simulink model "MultiBody2024bfinal"  (R2024b)
settings: Solver=ode45  StartTime=0.0  StopTime=5  FixedStep=0.001  RelTol=1e-3  AbsTol=1e-3  EnableMultiTasking=on
InitFcn:
  | contact_damping = 1e4;
  | contact_stiffness = 1e6;
values from neighbouring files (symbols this model uses):
  Angle = [30 30 0]    [main_SuperTwistingSMC2.m]
  Height = -(1.9 + i)    (= -5.9)    [main_SuperTwistingSMC2.m]
  i = 4    [main_SuperTwistingSMC2.m]
  nt = n_t(i)    [main_SuperTwistingSMC2.m]
  TM = TMM(i)    [main_SuperTwistingSMC2.m]
  TotalWeight = TotalWeightmb(i)    [main_SuperTwistingSMC2.m]
undefined symbols (not defined in the file or in its folder): X, Y, Z
libraries: sm_lib x207, nesl_utility x73, sharedtransform x6, simulink_extras x4
(part 7 of 7)

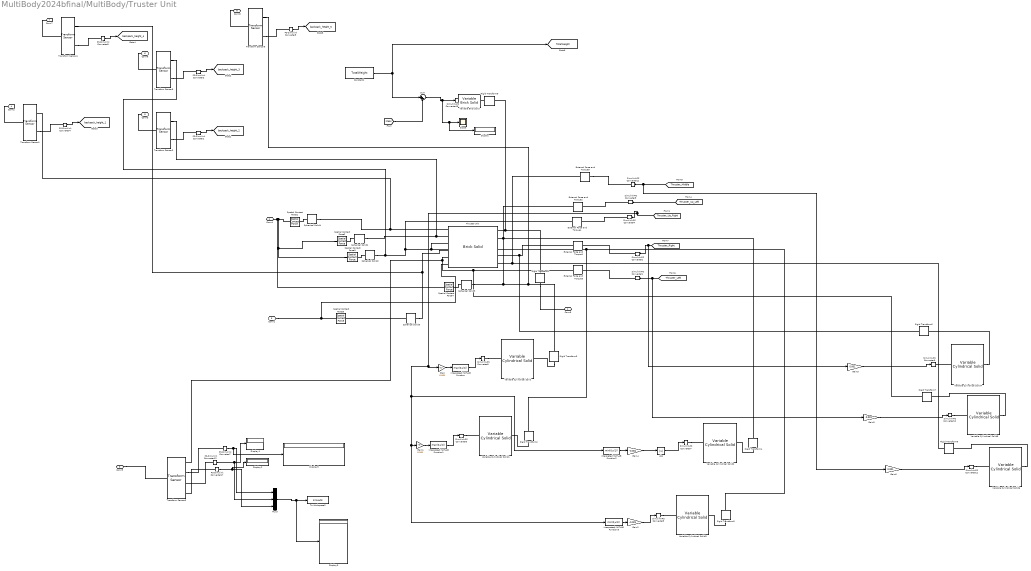
== system MultiBody2024bfinal/MultiBody/Truster Unit ==
  Abs : Abs  SaturateOnIntegerOverflow=off
  Constant1 : Constant  Value=TotalWeight
  Display{,1..3,5} (5 alike) : Display
  External Force and Torque1 : sm_lib/Forces and Torques/External Force and Torque  EnableForceX=off  EnableForceY=on  EnableForceZ=off  EnableForce=off  ForceResolutionFrame=AttachedFrame  EnableTorqueX=off  EnableTorqueY=off  EnableTorqueZ=off  EnableTorque=off  TorqueResolutionFrame=AttachedFrame
  External Force and Torque2 : sm_lib/Forces and Torques/External Force and Torque  EnableForceX=on  EnableForceY=off  EnableForceZ=off  EnableForce=off  ForceResolutionFrame=AttachedFrame  EnableTorqueX=off  EnableTorqueY=off  EnableTorqueZ=off  EnableTorque=off  TorqueResolutionFrame=AttachedFrame
  External Force and Torque3 : sm_lib/Forces and Torques/External Force and Torque  EnableForceX=off  EnableForceY=on  EnableForceZ=off  EnableForce=off  ForceResolutionFrame=AttachedFrame  EnableTorqueX=off  EnableTorqueY=off  EnableTorqueZ=off  EnableTorque=off  TorqueResolutionFrame=AttachedFrame
  External Force and Torque4 : sm_lib/Forces and Torques/External Force and Torque  EnableForceX=on  EnableForceY=off  EnableForceZ=off  EnableForce=off  ForceResolutionFrame=AttachedFrame  EnableTorqueX=off  EnableTorqueY=off  EnableTorqueZ=off  EnableTorque=off  TorqueResolutionFrame=AttachedFrame
  External Force and Torque5 : sm_lib/Forces and Torques/External Force and Torque  EnableForceX=off  EnableForceY=on  EnableForceZ=off  EnableForce=off  ForceResolutionFrame=AttachedFrame  EnableTorqueX=off  EnableTorqueY=off  EnableTorqueZ=off  EnableTorque=off  TorqueResolutionFrame=AttachedFrame
  Gain{,1,3,5..6} (5 alike) : Gain  Gain=0.001
  Gain2 : Gain  Gain=-0.001
  Gain4 : Gain  Gain=-0.001
  Interpreted MATLAB Function : MATLABFcn  MATLABFcn=max(0,u(1))
  Interpreted MATLAB Function1 : MATLABFcn  MATLABFcn=max(0,u(1))
  Interpreted MATLAB Function2 : MATLABFcn  MATLABFcn=min(0,u(1))
  Interpreted MATLAB Function3 : MATLABFcn  MATLABFcn=min(0,u(1))
  Mux3 : Mux  Inputs=3
  PS-Simulink Converter{1..5,7,12,17} (8 alike) : nesl_utility/PS-Simulink Converter  PhysicalDomain=network_engine_domain  SubClassName=ps_output  LeftPortType=input  RightPortType=output  PseudoPeriodic=off  Frequencies=[]  VectorFormat=inherit  Unit=inherit  AffineConversion=off
  Rigid Transform1 : sm_lib/Frames and Transforms/Rigid Transform  RotationMethod=None  FollAlignAxisA=+X  BaseAlignAxisA=+Y  FollAlignAxisB=+Y  BaseAlignAxisB=+Z  RotationStandardAxis=+Z  RotationAngle=0.0  RotationAngleUnits=deg  RotationArbitraryAxis=[0 0 1]  RotationSequenceAxes=FollowerAxes  RotationSequence=XYX  RotationSequenceAngles=[0 0 0]  RotationSequenceAnglesUnits=deg  RotationMatrix=[1 0 0; 0 1 0; 0 0 1]  Quaternion=[1 0 0 0]  TranslationMethod=Cartesian  TranslationCartesianOffset=[-0.17 0.17 1.903701373840161e-04]  TranslationCartesianOffsetUnits=m  TranslationStandardAxis=-X  TranslationStandardOffset=0.16  TranslationStandardOffsetUnits=m  TranslationROffset=0  TranslationROffsetUnits=m  TranslationThetaOffset=0  TranslationThetaOffsetUnits=deg  TranslationZOffset=0  TranslationZOffsetUnits=m
  Rigid Transform2 : sm_lib/Frames and Transforms/Rigid Transform  RotationMethod=StandardAxis  FollAlignAxisA=+X  BaseAlignAxisA=+Y  FollAlignAxisB=+Y  BaseAlignAxisB=+Z  RotationStandardAxis=+Y  RotationAngle=90  RotationAngleUnits=deg  RotationArbitraryAxis=[0 0 1]  RotationSequenceAxes=FollowerAxes  RotationSequence=XYX  RotationSequenceAngles=[0 0 0]  RotationSequenceAnglesUnits=deg  RotationMatrix=[1 0 0; 0 1 0; 0 0 1]  Quaternion=[1 0 0 0]  TranslationMethod=None  TranslationCartesianOffset=[-0.17 0.17 0]  TranslationCartesianOffsetUnits=m  TranslationStandardAxis=-X  TranslationStandardOffset=0.16  TranslationStandardOffsetUnits=m  TranslationROffset=0  TranslationROffsetUnits=m  TranslationThetaOffset=0  TranslationThetaOffsetUnits=deg  TranslationZOffset=0  TranslationZOffsetUnits=m
  Rigid Transform3 : sm_lib/Frames and Transforms/Rigid Transform  RotationMethod=StandardAxis  FollAlignAxisA=+X  BaseAlignAxisA=+Y  FollAlignAxisB=+Y  BaseAlignAxisB=+Z  RotationStandardAxis=+Y  RotationAngle=90  RotationAngleUnits=deg  RotationArbitraryAxis=[0 0 1]  RotationSequenceAxes=FollowerAxes  RotationSequence=XYX  RotationSequenceAngles=[0 0 0]  RotationSequenceAnglesUnits=deg  RotationMatrix=[1 0 0; 0 1 0; 0 0 1]  Quaternion=[1 0 0 0]  TranslationMethod=None  TranslationCartesianOffset=[-0.17 0.17 0]  TranslationCartesianOffsetUnits=m  TranslationStandardAxis=-X  TranslationStandardOffset=0.16  TranslationStandardOffsetUnits=m  TranslationROffset=0  TranslationROffsetUnits=m  TranslationThetaOffset=0  TranslationThetaOffsetUnits=deg  TranslationZOffset=0  TranslationZOffsetUnits=m
  Rigid Transform4 : sm_lib/Frames and Transforms/Rigid Transform  RotationMethod=StandardAxis  FollAlignAxisA=+X  BaseAlignAxisA=+Y  FollAlignAxisB=+Y  BaseAlignAxisB=+Z  RotationStandardAxis=+Y  RotationAngle=-90  RotationAngleUnits=deg  RotationArbitraryAxis=[0 0 1]  RotationSequenceAxes=FollowerAxes  RotationSequence=XYX  RotationSequenceAngles=[0 0 0]  RotationSequenceAnglesUnits=deg  RotationMatrix=[1 0 0; 0 1 0; 0 0 1]  Quaternion=[1 0 0 0]  TranslationMethod=None  TranslationCartesianOffset=[-0.17 0.17 0]  TranslationCartesianOffsetUnits=m  TranslationStandardAxis=-X  TranslationStandardOffset=0.16  TranslationStandardOffsetUnits=m  TranslationROffset=0  TranslationROffsetUnits=m  TranslationThetaOffset=0  TranslationThetaOffsetUnits=deg  TranslationZOffset=0  TranslationZOffsetUnits=m
  Rigid Transform5 : sm_lib/Frames and Transforms/Rigid Transform  RotationMethod=StandardAxis  FollAlignAxisA=+X  BaseAlignAxisA=+Y  FollAlignAxisB=+Y  BaseAlignAxisB=+Z  RotationStandardAxis=+Y  RotationAngle=-90  RotationAngleUnits=deg  RotationArbitraryAxis=[0 0 1]  RotationSequenceAxes=FollowerAxes  RotationSequence=XYX  RotationSequenceAngles=[0 0 0]  RotationSequenceAnglesUnits=deg  RotationMatrix=[1 0 0; 0 1 0; 0 0 1]  Quaternion=[1 0 0 0]  TranslationMethod=None  TranslationCartesianOffset=[-0.17 0.17 0]  TranslationCartesianOffsetUnits=m  TranslationStandardAxis=-X  TranslationStandardOffset=0.16  TranslationStandardOffsetUnits=m  TranslationROffset=0  TranslationROffsetUnits=m  TranslationThetaOffset=0  TranslationThetaOffsetUnits=deg  TranslationZOffset=0  TranslationZOffsetUnits=m
  Rigid Transform6 : sm_lib/Frames and Transforms/Rigid Transform  RotationMethod=StandardAxis  FollAlignAxisA=+X  BaseAlignAxisA=+Y  FollAlignAxisB=+Y  BaseAlignAxisB=+Z  RotationStandardAxis=+X  RotationAngle=-90  RotationAngleUnits=deg  RotationArbitraryAxis=[0 0 1]  RotationSequenceAxes=FollowerAxes  RotationSequence=XYX  RotationSequenceAngles=[0 0 0]  RotationSequenceAnglesUnits=deg  RotationMatrix=[1 0 0; 0 1 0; 0 0 1]  Quaternion=[1 0 0 0]  TranslationMethod=None  TranslationCartesianOffset=[-0.17 0.17 0]  TranslationCartesianOffsetUnits=m  TranslationStandardAxis=-X  TranslationStandardOffset=0.16  TranslationStandardOffsetUnits=m  TranslationROffset=0  TranslationROffsetUnits=m  TranslationThetaOffset=0  TranslationThetaOffsetUnits=deg  TranslationZOffset=0  TranslationZOffsetUnits=m
  Rigid Transform7 : sm_lib/Frames and Transforms/Rigid Transform  RotationMethod=StandardAxis  FollAlignAxisA=+X  BaseAlignAxisA=+Y  FollAlignAxisB=+Y  BaseAlignAxisB=+Z  RotationStandardAxis=+X  RotationAngle=-90  RotationAngleUnits=deg  RotationArbitraryAxis=[0 0 1]  RotationSequenceAxes=FollowerAxes  RotationSequence=XYX  RotationSequenceAngles=[0 0 0]  RotationSequenceAnglesUnits=deg  RotationMatrix=[1 0 0; 0 1 0; 0 0 1]  Quaternion=[1 0 0 0]  TranslationMethod=None  TranslationCartesianOffset=[-0.17 0.17 0]  TranslationCartesianOffsetUnits=m  TranslationStandardAxis=-X  TranslationStandardOffset=0.16  TranslationStandardOffsetUnits=m  TranslationROffset=0  TranslationROffsetUnits=m  TranslationThetaOffset=0  TranslationThetaOffsetUnits=deg  TranslationZOffset=0  TranslationZOffsetUnits=m
  Rigid Transform8 : sm_lib/Frames and Transforms/Rigid Transform  RotationMethod=StandardAxis  FollAlignAxisA=+X  BaseAlignAxisA=+Y  FollAlignAxisB=+Y  BaseAlignAxisB=+Z  RotationStandardAxis=+X  RotationAngle=-90  RotationAngleUnits=deg  RotationArbitraryAxis=[0 0 1]  RotationSequenceAxes=FollowerAxes  RotationSequence=XYX  RotationSequenceAngles=[0 0 0]  RotationSequenceAnglesUnits=deg  RotationMatrix=[1 0 0; 0 1 0; 0 0 1]  Quaternion=[1 0 0 0]  TranslationMethod=None  TranslationCartesianOffset=[-0.17 0.17 0]  TranslationCartesianOffsetUnits=m  TranslationStandardAxis=-X  TranslationStandardOffset=0.16  TranslationStandardOffsetUnits=m  TranslationROffset=0  TranslationROffsetUnits=m  TranslationThetaOffset=0  TranslationThetaOffsetUnits=deg  TranslationZOffset=0  TranslationZOffsetUnits=m
  Rigid Transform9 : sm_lib/Frames and Transforms/Rigid Transform  RotationMethod=None  FollAlignAxisA=+X  BaseAlignAxisA=+Y  FollAlignAxisB=+Y  BaseAlignAxisB=+Z  RotationStandardAxis=+Z  RotationAngle=0.0  RotationAngleUnits=deg  RotationArbitraryAxis=[0 0 1]  RotationSequenceAxes=FollowerAxes  RotationSequence=XYX  RotationSequenceAngles=[0 0 0]  RotationSequenceAnglesUnits=deg  RotationMatrix=[1 0 0; 0 1 0; 0 0 1]  Quaternion=[1 0 0 0]  TranslationMethod=Cartesian  TranslationCartesianOffset=[0 0 -0.33/2]  TranslationCartesianOffsetUnits=m  TranslationStandardAxis=-X  TranslationStandardOffset=0.16  TranslationStandardOffsetUnits=m  TranslationROffset=0  TranslationROffsetUnits=m  TranslationThetaOffset=0  TranslationThetaOffsetUnits=deg  TranslationZOffset=0  TranslationZOffsetUnits=m
  Scope : Scope
  Simulink-PS Converter{1..13} (13 alike) : nesl_utility/Simulink-PS Converter  PhysicalDomain=network_engine_domain  SubClassName=ps_input  LeftPortType=input  RightPortType=output  PseudoPeriodic=off  Frequencies=[]  NoiseDistribution=none  NoiseParameters=[]  Unit=1  AffineConversion=off  FilteringAndDerivatives=provide  SimscapeFilterOrder=1  InputFilterTimeConstant=0.001  UdotUserProvided=0
  Spatial Contact Force{1..5} (5 alike) : sm_lib/Forces and Torques/Spatial Contact Force  NormalForceType=SmoothSpringDamper  NormalStiffness=contact_stiffness  NormalStiffnessUnits=N/m  NormalDamping=contact_damping  NormalDampingUnits=N/(m/s)  NormalTransitionRegionWidth=1e-4  NormalTransitionRegionWidthUnits=m  FrictionType=SmoothStickSlip  CoefficientOfStaticFriction=0.5  CoefficientOfDynamicFriction=0.3  FrictionalCriticalVelocity=1e-3  FrictionalCriticalVelocityUnits=m/s  SenseContactSignal=off  SensePenetrationDepth=off  SenseSeparationDistance=off  SenseNormalForceMagnitude=off  SenseFrictionalForceMagnitude=off  SenseNormalVelocity=off  SenseTangentialVelocity=off  SenseContactBaseRotation=off  SenseContactBaseTranslation=off  SenseContactFollowerRotation=off  SenseContactFollowerTranslation=off  ZeroCrossDetectContactStartAndEnd=off
  Spherical Solid{1..5} (5 alike) : sm_lib/Body Elements/Spherical Solid  SphereRadius=0.01  SphereRadiusUnits=m  ExportEntireGeometry=on  InertiaType=CalculateFromGeometry  BasedOnType=Density  Density=0  DensityUnits=kg/m^3  Mass=1  MassUnits=kg  CenterOfMass=[0 0 0]  CenterOfMassUnits=m  MomentsOfInertia=[1 1 1]  MomentsOfInertiaUnits=kg*m^2  ProductsOfInertia=[0 0 0]  ProductsOfInertiaUnits=kg*m^2  GraphicType=None  MarkerShape=Sphere  MarkerSize=10  GraphicVisPropType=SimpleVisualProperties  GraphicDiffuseColor=[1.0 0.0 0.0]  GraphicOpacity=1.0  GraphicSpecularColor=[0.5 0.5 0.5 1.0]  GraphicAmbientColor=[0.15 0.15 0.15 1.0]  GraphicEmissiveColor=[0.0 0.0 0.0 1.0]  GraphicShininess=75  DoExposeReferenceFrame=on  SerializedFrames=<Frames/>
  Sum : Sum  Inputs=|+-
  Thruster Unit : sm_lib/Body Elements/Brick Solid  BrickDimensions=[0.12 0.52 0.33]  BrickDimensionsUnits=m  ExportEntireGeometry=on  InertiaType=CalculateFromGeometry  BasedOnType=Mass  Density=1000  DensityUnits=kg/m^3  Mass=0.001  MassUnits=kg  CenterOfMass=[0 0 0]  CenterOfMassUnits=m  MomentsOfInertia=[1 1 1]  MomentsOfInertiaUnits=kg*m^2  ProductsOfInertia=[0 0 0]  ProductsOfInertiaUnits=kg*m^2  GraphicType=FromGeometry  MarkerShape=Sphere  MarkerSize=10  GraphicVisPropType=SimpleVisualProperties  GraphicDiffuseColor=[0.0 1.0 0.0]  GraphicOpacity=1.0  GraphicSpecularColor=[0.5 0.5 0.5 1.0]  GraphicAmbientColor=[0.15 0.15 0.15 1.0]  GraphicEmissiveColor=[0.0 0.0 0.0 1.0]  GraphicShininess=75  DoExposeReferenceFrame=on  SerializedFrames=<Frames><Frame><Id>Frame1</Id><Value><Name>F1</Name><Origin><Source>GeometricFeature</Source><FeatureName>-x -y +z point</FeatureName></Origin><PrimaryAxis><DefinedDirection>+Z</DefinedDirection><Source>ReferenceFrame</Source><SourceDirection>+Z</SourceDirection><FeatureName></FeatureName></PrimaryAxis><SecondaryAxis><DefinedDirection>+X</DefinedDirection><Source>ReferenceFrame</Source><SourceDirection>+X</SourceDirection><FeatureName></FeatureName></SecondaryAxis></Value></Frame><Frame><Id>Frame2</Id><Value><Name>F2</Name><Origin><Source>GeometricFeature</Source><FeatureName>-x -y -z point</FeatureName></Origin><PrimaryAxis><DefinedDirection>+Z</DefinedDirection><Source>ReferenceFrame</Source><SourceDirection>+Z</SourceDirection><FeatureName></FeatureName></PrimaryAxis><SecondaryAxis><DefinedDirection>+X</DefinedDirection><Source>ReferenceFrame</Source><SourceDirection>+X</SourceDirection><FeatureName></FeatureName></SecondaryAxis></Value></Frame><Frame><Id>Frame3</Id><Value><Name>Thruster_3</Name><Origin><Source>GeometricFeature</Source><FeatureName>-x +y -z point</FeatureName></Origin><PrimaryAxis><DefinedDirection>+Z</DefinedDirection><Source>ReferenceFrame</Source><SourceDirection>+Z</SourceDirection><FeatureName></FeatureName></PrimaryAxis><SecondaryAxis><DefinedDirection>+X</DefinedDirection><Source>ReferenceFrame</Source><SourceDirection>+X</SourceDirection><FeatureName></FeatureName></SecondaryAxis></Value></Frame><Frame><Id>Frame4</Id><Value><Name>Thruster_4</Name><Origin><Source>GeometricFeature</Source><FeatureName>-x +y +z point</FeatureName></Origin><PrimaryAxis><DefinedDirection>+Z</DefinedDirection><Source>ReferenceFrame</Source><SourceDirection>+Z</SourceDirection><FeatureName></FeatureName></PrimaryAxis><SecondaryAxis><DefinedDirection>+X</DefinedDirection><Source>ReferenceFrame</Source><SourceDirection>+X</SourceDirection><FeatureName></FeatureName></SecondaryAxis></Value></Frame><Frame><Id>Frame5</Id><Value><Name>F5</Name><Origin><Source>GeometricFeature</Source><FeatureName>+x -y curve</FeatureName></Origin><PrimaryAxis><DefinedDirection>+Z</DefinedDirection><Source>ReferenceFrame</Source><SourceDirection>+Z</SourceDirection><FeatureName></FeatureName></PrimaryAxis><SecondaryAxis><DefinedDirection>+X</DefinedDirection><Source>ReferenceFrame</Source><SourceDirection>+X</SourceDirection><FeatureName></FeatureName></SecondaryAxis></Value></Frame><Frame><Id>Frame6</Id><Value><Name>F6</Name><Origin><Source>GeometricFeature</Source><FeatureName>+z +x curve</FeatureName></Origin><PrimaryAxis><DefinedDirection>+Z</DefinedDirection><Source>ReferenceFrame</Source><SourceDirection>+Z</SourceDirection><FeatureName></FeatureName></PrimaryAxis><SecondaryAxis><DefinedDirection>+X</DefinedDirection><Source>ReferenceFrame</Source><SourceDirection>+X</SourceDirection><FeatureName></FeatureName></SecondaryAxis></Value></Frame><Frame><Id>Frame7</Id><Value><Name>Thruster_1</Name><Origin><Source>GeometricFeature</Source><FeatureName>-y +z curve</FeatureName></Origin><PrimaryAxis><DefinedDirection>+Z</DefinedDirection><Source>ReferenceFrame</Source><SourceDirection>+Z</SourceDirection><FeatureName></FeatureName></PrimaryAxis><SecondaryAxis><DefinedDirection>+X</DefinedDirection><Source>ReferenceFrame</Source><SourceDirection>+X</SourceDirection><FeatureName></FeatureName></SecondaryAxis></Value></Frame><Frame><Id>Frame8</Id><Value><Name>Thruster_2</Name><Origin><Source>GeometricFeature</Source><FeatureName>-y -z curve</FeatureName></Origin><PrimaryAxis><DefinedDirection>+Z</DefinedDirection><Source>ReferenceFrame</Source><SourceDirection>+Z</SourceDirection><FeatureName></FeatureName></PrimaryAxis><SecondaryAxis><DefinedDirection>+X</DefinedDirection><Source>ReferenceFrame</Source><SourceDirection>+X</SourceDirection><FeatureName></FeatureName></SecondaryAxis></Value></Frame><Frame><Id>Frame9</Id><Value><Name>Thruster_0</Name><Origin><Source>GeometricFeature</Source><FeatureName>-y surface</FeatureName></Origin><PrimaryAxis><DefinedDirection>+Z</DefinedDirection><Source>ReferenceFrame</Source><SourceDirection>+Z</SourceDirection><FeatureName></FeatureName></PrimaryAxis><SecondaryAxis><DefinedDirection>+X</DefinedDirection><Source>ReferenceFrame</Source><SourceDirection>+X</SourceDirection><FeatureName></FeatureName></SecondaryAxis></Value></Frame></Frames>
  To Workspace2 : ToWorkspace  VariableName=simout3  SampleTime=-1
      settings: Save2DSignal=2-D array (concatenate along first dimension)
  Transform Sensor{1..5} (5 alike) : sm_lib/Frames and Transforms/Transform Sensor  MeasurementFrame=World  RotationSequence=XYX  SenseAngle=off  SenseAxis=off  SenseQ=off  SenseR=off  SenseRotationSequence=off  SenseOmegaX=off  SenseOmegaY=off  SenseOmegaZ=off  SenseOmega=off  SenseQDot=off  SenseRDot=off  SenseRotationSequenceDot=off  SenseAlphaX=off  SenseAlphaY=off  SenseAlphaZ=off  SenseAlpha=off  SenseQDDot=off  SenseRDDot=off  SenseX=off  SenseY=off  SenseZ=on  SenseXYZ=off  SenseRad=off  SenseAzim=off  SenseDist=off  SenseInc=off  SenseXDot=off  SenseYDot=off  SenseZDot=off  SenseXYZDot=off  SenseRadDot=off  SenseAzimDot=off  SenseDistDot=off  SenseIncDot=off  SenseXDDot=off  SenseYDDot=off  SenseZDDot=off  SenseXYZDDot=off  SenseRadDDot=off  SenseAzimDDot=off  SenseDistDDot=off  SenseIncDDot=off
  Transform Sensor6 : sm_lib/Frames and Transforms/Transform Sensor  MeasurementFrame=Base  RotationSequence=XYZ  SenseAngle=off  SenseAxis=off  SenseQ=off  SenseR=off  SenseRotationSequence=off  SenseOmegaX=off  SenseOmegaY=off  SenseOmegaZ=off  SenseOmega=off  SenseQDot=off  SenseRDot=off  SenseRotationSequenceDot=off  SenseAlphaX=off  SenseAlphaY=off  SenseAlphaZ=off  SenseAlpha=off  SenseQDDot=off  SenseRDDot=off  SenseX=on  SenseY=on  SenseZ=on  SenseXYZ=off  SenseRad=off  SenseAzim=off  SenseDist=off  SenseInc=off  SenseXDot=off  SenseYDot=off  SenseZDot=off  SenseXYZDot=off  SenseRadDot=off  SenseAzimDot=off  SenseDistDot=off  SenseIncDot=off  SenseXDDot=off  SenseYDDot=off  SenseZDDot=off  SenseXYZDDot=off  SenseRadDDot=off  SenseAzimDDot=off  SenseDistDDot=off  SenseIncDDot=off
  Variable Brick Solid : sm_lib/Body Elements/Variable Mass/Variable Brick Solid  XLengthType=Constant  XLength=0.115  XLengthUnits=m  YLengthType=Constant  YLength=0.515  YLengthUnits=m  ZLengthType=Constant  ZLength=0.325  ZLengthUnits=m  MassType=ProvidedByInput  Density=1000  DensityUnits=kg/m^3  SenseXLength=off  SenseYLength=off  SenseZLength=off  SenseMass=off  SenseCenterOfMass=off  SenseInertiaMatrix=off  GraphicType=FromGeometry  MarkerShape=Sphere  MarkerSize=10  GraphicVisPropType=SimpleVisualProperties  GraphicDiffuseColor=[0 1 0]  GraphicOpacity=1.0  GraphicSpecularColor=[0.5 0.5 0.5 1.0]  GraphicAmbientColor=[0.15 0.15 0.15 1.0]  GraphicEmissiveColor=[0.0 0.0 0.0 1.0]  GraphicShininess=75
  Variable Cylindrical Solid : sm_lib/Body Elements/Variable Mass/Variable Cylindrical Solid  RadiusType=Constant  Radius=0.01  RadiusUnits=m  LengthType=ProvidedByInput  Length=1  LengthUnits=m  MassType=CalculateFromGeometry  Density=0.0000000001  DensityUnits=kg/m^3  SenseRadius=off  SenseLength=off  SenseMass=off  SenseCenterOfMass=off  SenseInertiaMatrix=off  GraphicType=FromGeometry  MarkerShape=Cube  MarkerSize=10  GraphicVisPropType=SimpleVisualProperties  GraphicDiffuseColor=[1 0 0]  GraphicOpacity=1.0  GraphicSpecularColor=[0.5 0.5 0.5 1.0]  GraphicAmbientColor=[0.15 0.15 0.15 1.0]  GraphicEmissiveColor=[0.0 0.0 0.0 1.0]  GraphicShininess=75
  Variable Cylindrical Solid1 : sm_lib/Body Elements/Variable Mass/Variable Cylindrical Solid  RadiusType=Constant  Radius=0.01  RadiusUnits=m  LengthType=ProvidedByInput  Length=1  LengthUnits=m  MassType=CalculateFromGeometry  Density=0.0000000001  DensityUnits=kg/m^3  SenseRadius=off  SenseLength=off  SenseMass=off  SenseCenterOfMass=off  SenseInertiaMatrix=off  GraphicType=FromGeometry  MarkerShape=Cube  MarkerSize=10  GraphicVisPropType=SimpleVisualProperties  GraphicDiffuseColor=[1 0 0]  GraphicOpacity=1.0  GraphicSpecularColor=[0.5 0.5 0.5 1.0]  GraphicAmbientColor=[0.15 0.15 0.15 1.0]  GraphicEmissiveColor=[0.0 0.0 0.0 1.0]  GraphicShininess=75
  Variable Cylindrical Solid2 : sm_lib/Body Elements/Variable Mass/Variable Cylindrical Solid  RadiusType=Constant  Radius=0.01  RadiusUnits=m  LengthType=ProvidedByInput  Length=1  LengthUnits=m  MassType=CalculateFromGeometry  Density=0.0000000001  DensityUnits=kg/m^3  SenseRadius=off  SenseLength=off  SenseMass=off  SenseCenterOfMass=off  SenseInertiaMatrix=off  GraphicType=FromGeometry  MarkerShape=Cube  MarkerSize=10  GraphicVisPropType=SimpleVisualProperties  GraphicDiffuseColor=[0 0 1]  GraphicOpacity=1.0  GraphicSpecularColor=[0.5 0.5 0.5 1.0]  GraphicAmbientColor=[0.15 0.15 0.15 1.0]  GraphicEmissiveColor=[0.0 0.0 0.0 1.0]  GraphicShininess=75
  Variable Cylindrical Solid3 : sm_lib/Body Elements/Variable Mass/Variable Cylindrical Solid  RadiusType=Constant  Radius=0.01  RadiusUnits=m  LengthType=ProvidedByInput  Length=1  LengthUnits=m  MassType=CalculateFromGeometry  Density=0.0000000001  DensityUnits=kg/m^3  SenseRadius=off  SenseLength=off  SenseMass=off  SenseCenterOfMass=off  SenseInertiaMatrix=off  GraphicType=FromGeometry  MarkerShape=Cube  MarkerSize=10  GraphicVisPropType=SimpleVisualProperties  GraphicDiffuseColor=[0 0 1]  GraphicOpacity=1.0  GraphicSpecularColor=[0.5 0.5 0.5 1.0]  GraphicAmbientColor=[0.15 0.15 0.15 1.0]  GraphicEmissiveColor=[0.0 0.0 0.0 1.0]  GraphicShininess=75
  Variable Cylindrical Solid4 : sm_lib/Body Elements/Variable Mass/Variable Cylindrical Solid  RadiusType=Constant  Radius=0.01  RadiusUnits=m  LengthType=ProvidedByInput  Length=1  LengthUnits=m  MassType=CalculateFromGeometry  Density=0.0000000001  DensityUnits=kg/m^3  SenseRadius=off  SenseLength=off  SenseMass=off  SenseCenterOfMass=off  SenseInertiaMatrix=off  GraphicType=FromGeometry  MarkerShape=Cube  MarkerSize=10  GraphicVisPropType=SimpleVisualProperties  GraphicDiffuseColor=[1 0 1]  GraphicOpacity=1.0  GraphicSpecularColor=[0.5 0.5 0.5 1.0]  GraphicAmbientColor=[0.15 0.15 0.15 1.0]  GraphicEmissiveColor=[0.0 0.0 0.0 1.0]  GraphicShininess=75
  Variable Cylindrical Solid5 : sm_lib/Body Elements/Variable Mass/Variable Cylindrical Solid  RadiusType=Constant  Radius=0.01  RadiusUnits=m  LengthType=ProvidedByInput  Length=1  LengthUnits=m  MassType=CalculateFromGeometry  Density=0.0000000001  DensityUnits=kg/m^3  SenseRadius=off  SenseLength=off  SenseMass=off  SenseCenterOfMass=off  SenseInertiaMatrix=off  GraphicType=FromGeometry  MarkerShape=Cube  MarkerSize=10  GraphicVisPropType=SimpleVisualProperties  GraphicDiffuseColor=[1 0 1]  GraphicOpacity=1.0  GraphicSpecularColor=[0.5 0.5 0.5 1.0]  GraphicAmbientColor=[0.15 0.15 0.15 1.0]  GraphicEmissiveColor=[0.0 0.0 0.0 1.0]  GraphicShininess=75
  Variable Cylindrical Solid6 : sm_lib/Body Elements/Variable Mass/Variable Cylindrical Solid  RadiusType=Constant  Radius=0.01  RadiusUnits=m  LengthType=ProvidedByInput  Length=1  LengthUnits=m  MassType=CalculateFromGeometry  Density=0.0000000001  DensityUnits=kg/m^3  SenseRadius=off  SenseLength=off  SenseMass=off  SenseCenterOfMass=off  SenseInertiaMatrix=off  GraphicType=FromGeometry  MarkerShape=Cube  MarkerSize=10  GraphicVisPropType=SimpleVisualProperties  GraphicDiffuseColor=[1 0 1]  GraphicOpacity=1.0  GraphicSpecularColor=[0.5 0.5 0.5 1.0]  GraphicAmbientColor=[0.15 0.15 0.15 1.0]  GraphicEmissiveColor=[0.0 0.0 0.0 1.0]  GraphicShininess=75
  Conn5 : PMIOPort  Side=Left
  Conn4 : PMIOPort  Port=2  Side=Left
  Conn1 : PMIOPort  Port=3  Side=Left
  Conn2 : PMIOPort  Port=4  Side=Left
  Conn3 : PMIOPort  Port=5  Side=Left
  Conn6 : PMIOPort  Port=6  Side=Left
  Conn7 : PMIOPort  Port=7  Side=Left
  Conn8 : PMIOPort  Port=8  Side=Left
  Conn9 : PMIOPort  Port=9  Side=Left
  tag scope: TotalWeight=global, backpack_height_1=global, backpack_height_2=global, backpack_height_3=global, backpack_height_4=global, backpack_height_5=global
  wires:
  Gain/1 -> Interpreted MATLAB Function/1
  Interpreted MATLAB Function/1 -> Simulink-PS Converter5/1
  Interpreted MATLAB Function1/1 -> Simulink-PS Converter6/1
  Gain1/1 -> Interpreted MATLAB Function1/1
  Interpreted MATLAB Function2/1 -> Gain4/1
  Interpreted MATLAB Function3/1 -> Gain2/1
  [Thruster_Up_Right] -> Simulink-PS Converter4/1, Interpreted MATLAB Function2/1, Interpreted MATLAB Function3/1, Gain1/1, Gain/1
  Gain4/1 -> Abs/1
  Gain2/1 -> Simulink-PS Converter8/1
  Gain3/1 -> Simulink-PS Converter9/1
  [Thruster_Right] -> Gain3/1, Simulink-PS Converter2/1
  [Thruster_Left] -> Gain5/1, Simulink-PS Converter1/1
  Gain5/1 -> Simulink-PS Converter10/1
  Gain6/1 -> Simulink-PS Converter12/1
  [Thruster_Middle] -> Gain6/1, Simulink-PS Converter11/1
  Abs/1 -> Simulink-PS Converter7/1
  PS-Simulink Converter4/1 -> [backpack_height_1]
  PS-Simulink Converter1/1 -> [backpack_height_2]
  PS-Simulink Converter2/1 -> [backpack_height_3]
  PS-Simulink Converter3/1 -> [backpack_height_4]
  PS-Simulink Converter5/1 -> [backpack_height_5]
  Sum/1 -> Display/1, Scope/1, Simulink-PS Converter13/1
  [Mass] -> Sum/2
  Constant1/1 -> [TotalWeight], Sum/1
  [Thruster_Up_Left] -> Simulink-PS Converter3/1
  PS-Simulink Converter7/1 -> Mux3/1, Display5/1
  Mux3/1 -> Display3/1, To Workspace2/1
  PS-Simulink Converter17/1 -> Mux3/3, Display2/1
  PS-Simulink Converter12/1 -> Mux3/2, Display1/1
  connections:
  Rigid Transform1/RConn1 -- Rigid Transform9/LConn1 -- Thruster Unit/RConn1
  Rigid Transform1/LConn1 -- Conn5/RConn1
  Simulink-PS Converter2/RConn1 -- External Force and Torque1/LConn1
  Simulink-PS Converter1/RConn1 -- External Force and Torque3/LConn1
  Simulink-PS Converter4/RConn1 -- External Force and Torque4/LConn1
  Spatial Contact Force1/RConn1 -- Spatial Contact Force2/RConn1 -- Spatial Contact Force3/RConn1 -- Spatial Contact Force4/RConn1 -- Conn4/RConn1
  Spherical Solid4/LConn1 -- Spatial Contact Force1/LConn1
  Spherical Solid4/RConn1 -- Transform Sensor1/RConn1 -- Thruster Unit/LConn1
  Spherical Solid1/LConn1 -- Spatial Contact Force2/LConn1
  Spherical Solid1/RConn1 -- Thruster Unit/LConn2 -- Transform Sensor2/RConn1
  Spherical Solid2/LConn1 -- Spatial Contact Force3/LConn1
  Spherical Solid2/RConn1 -- Transform Sensor3/RConn1 -- External Force and Torque4/RConn1 -- Rigid Transform5/RConn1 -- Rigid Transform2/RConn1 -- Thruster Unit/LConn3
  Spherical Solid3/LConn1 -- Spatial Contact Force4/LConn1
  Conn1/RConn1 -- Thruster Unit/LConn6 -- Spatial Contact Force5/RConn1
  Spherical Solid5/RConn1 -- Transform Sensor4/RConn1 -- Thruster Unit/LConn4
  Spherical Solid5/LConn1 -- Spatial Contact Force5/LConn1
  External Force and Torque1/RConn1 -- Rigid Transform6/RConn1 -- Thruster Unit/RConn4
  External Force and Torque3/RConn1 -- Transform Sensor6/RConn1 -- Thruster Unit/LConn5 -- Rigid Transform7/RConn1
  Simulink-PS Converter3/RConn1 -- External Force and Torque2/LConn1
  Simulink-PS Converter5/RConn1 -- Variable Cylindrical Solid/LConn1
  Rigid Transform3/LConn1 -- Variable Cylindrical Solid/RConn1
  External Force and Torque2/RConn1 -- Rigid Transform4/RConn1 -- Spherical Solid3/RConn1 -- Rigid Transform3/RConn1 -- Transform Sensor5/RConn1 -- Thruster Unit/RConn2
  Rigid Transform2/LConn1 -- Variable Cylindrical Solid1/RConn1
  Simulink-PS Converter6/RConn1 -- Variable Cylindrical Solid1/LConn1
  Simulink-PS Converter7/RConn1 -- Variable Cylindrical Solid2/LConn1
  Rigid Transform4/LConn1 -- Variable Cylindrical Solid2/RConn1
  Rigid Transform5/LConn1 -- Variable Cylindrical Solid3/RConn1
  Simulink-PS Converter8/RConn1 -- Variable Cylindrical Solid3/LConn1
  Simulink-PS Converter9/RConn1 -- Variable Cylindrical Solid4/LConn1
  Variable Cylindrical Solid4/RConn1 -- Rigid Transform6/LConn1
  Variable Cylindrical Solid5/RConn1 -- Rigid Transform7/LConn1
  Simulink-PS Converter10/RConn1 -- Variable Cylindrical Solid5/LConn1
  External Force and Torque5/RConn1 -- Thruster Unit/RConn5 -- Rigid Transform8/RConn1
  External Force and Torque5/LConn1 -- Simulink-PS Converter11/RConn1
  Simulink-PS Converter12/RConn1 -- Variable Cylindrical Solid6/LConn1
  Variable Cylindrical Solid6/RConn1 -- Rigid Transform8/LConn1
  Transform Sensor1/RConn2 -- PS-Simulink Converter4/LConn1
  Transform Sensor1/LConn1 -- Conn2/RConn1
  Transform Sensor2/LConn1 -- Conn3/RConn1
  Transform Sensor2/RConn2 -- PS-Simulink Converter1/LConn1
  Transform Sensor3/RConn2 -- PS-Simulink Converter2/LConn1
  Transform Sensor3/LConn1 -- Conn6/RConn1
  Transform Sensor4/LConn1 -- Conn7/RConn1
  Transform Sensor4/RConn2 -- PS-Simulink Converter3/LConn1
  Transform Sensor5/RConn2 -- PS-Simulink Converter5/LConn1
  Transform Sensor5/LConn1 -- Conn8/RConn1
  Simulink-PS Converter13/RConn1 -- Variable Brick Solid/LConn1
  Rigid Transform9/RConn1 -- Variable Brick Solid/RConn1
  Transform Sensor6/RConn2 -- PS-Simulink Converter7/LConn1
  Conn9/RConn1 -- Transform Sensor6/LConn1
  PS-Simulink Converter17/LConn1 -- Transform Sensor6/RConn4
  PS-Simulink Converter12/LConn1 -- Transform Sensor6/RConn3

== system MultiBody2024bfinal/Super Twisting Sliding Mode Controller/PWPF1 ==
  In1 : Inport
  Relay2 : Relay  OnSwitchValue=Uon  OffSwitchValue=Uoff  OnOutputValue=Um
  Relay3 : Relay  OnSwitchValue=-Uoff  OffSwitchValue=-Uon  OnOutputValue=0  OffOutputValue=-Um
  Sum1 : Sum
  Sum3 : Sum  Inputs=|+-
  Transfer Fcn9 : TransferFcn  Numerator=Km  Denominator=[Tm 1]
  Thrust : Outport
  wires:
  Transfer Fcn9/1 -> Relay2/1, Relay3/1
  Relay3/1 -> Sum1/2
  Relay2/1 -> Sum1/1
  Sum1/1 -> Thrust/1, Sum3/2
  In1/1 -> Sum3/1
  Sum3/1 -> Transfer Fcn9/1

== system MultiBody2024bfinal/Super Twisting Sliding Mode Controller/PWPF2 ==
  In1 : Inport
  Relay2 : Relay  OnSwitchValue=Uon  OffSwitchValue=Uoff  OnOutputValue=Um
  Relay3 : Relay  OnSwitchValue=-Uoff  OffSwitchValue=-Uon  OnOutputValue=0  OffOutputValue=-Um
  Sum1 : Sum
  Sum3 : Sum  Inputs=|+-
  Transfer Fcn9 : TransferFcn  Numerator=Km  Denominator=[Tm 1]
  Thrust : Outport
  wires:
  Sum3/1 -> Transfer Fcn9/1
  In1/1 -> Sum3/1
  Sum1/1 -> Sum3/2, Thrust/1
  Relay2/1 -> Sum1/1
  Relay3/1 -> Sum1/2
  Transfer Fcn9/1 -> Relay3/1, Relay2/1

== system MultiBody2024bfinal/Super Twisting Sliding Mode Controller/PWPF3 ==
  In1 : Inport
  Relay2 : Relay  OnSwitchValue=Uon  OffSwitchValue=Uoff  OnOutputValue=Um
  Relay3 : Relay  OnSwitchValue=-Uoff  OffSwitchValue=-Uon  OnOutputValue=0  OffOutputValue=-Um
  Sum1 : Sum
  Sum3 : Sum  Inputs=|+-
  Transfer Fcn9 : TransferFcn  Numerator=Km  Denominator=[Tm 1]
  Thrust : Outport
  wires:
  Transfer Fcn9/1 -> Relay2/1, Relay3/1
  Relay3/1 -> Sum1/2
  Relay2/1 -> Sum1/1
  Sum1/1 -> Thrust/1, Sum3/2
  In1/1 -> Sum3/1
  Sum3/1 -> Transfer Fcn9/1

== system MultiBody2024bfinal/Super Twisting Sliding Mode Controller/PWPF4 ==
  In1 : Inport
  Relay2 : Relay  OnSwitchValue=Uon  OffSwitchValue=Uoff  OnOutputValue=Um
  Relay3 : Relay  OnSwitchValue=-Uoff  OffSwitchValue=-Uon  OnOutputValue=0  OffOutputValue=-Um
  Sum1 : Sum
  Sum3 : Sum  Inputs=|+-
  Transfer Fcn9 : TransferFcn  Numerator=Km  Denominator=[Tm 1]
  Thrust : Outport
  wires:
  Sum3/1 -> Transfer Fcn9/1
  In1/1 -> Sum3/1
  Sum1/1 -> Sum3/2, Thrust/1
  Relay2/1 -> Sum1/1
  Relay3/1 -> Sum1/2
  Transfer Fcn9/1 -> Relay3/1, Relay2/1

== system MultiBody2024bfinal/Super Twisting Sliding Mode Controller/PWPF5 ==
  In1 : Inport
  Relay2 : Relay  OnSwitchValue=Uon  OffSwitchValue=Uoff  OnOutputValue=Um
  Relay3 : Relay  OnSwitchValue=-Uoff  OffSwitchValue=-Uon  OnOutputValue=0  OffOutputValue=-Um
  Sum1 : Sum
  Sum3 : Sum  Inputs=|+-
  Transfer Fcn9 : TransferFcn  Numerator=Km  Denominator=[Tm 1]
  Thrust : Outport
  wires:
  Transfer Fcn9/1 -> Relay2/1, Relay3/1
  Relay3/1 -> Sum1/2
  Relay2/1 -> Sum1/1
  Sum1/1 -> Thrust/1, Sum3/2
  In1/1 -> Sum3/1
  Sum3/1 -> Transfer Fcn9/1

== system MultiBody2024bfinal/Super Twisting Sliding Mode Controller/unwrap1 ==
  input_angle : Inport
  MATLAB Function1 : MATLAB Function  TreatAsAtomicUnit=on
  Memory : Memory
  unwrapped_angle : Outport
  wires:
  input_angle/1 -> MATLAB Function1/1(input_angle)
  Memory/1 -> MATLAB Function1/2(prev_angle)
  MATLAB Function1/1(unwrapped_angle) -> Memory/1, unwrapped_angle/1

== system MultiBody2024bfinal/Super Twisting Sliding Mode Controller/unwrap2 ==
  input_angle : Inport
  MATLAB Function1 : MATLAB Function  TreatAsAtomicUnit=on
  Memory : Memory
  unwrapped_angle : Outport
  wires:
  MATLAB Function1/1(unwrapped_angle) -> unwrapped_angle/1, Memory/1
  Memory/1 -> MATLAB Function1/2(prev_angle)
  input_angle/1 -> MATLAB Function1/1(input_angle)

== system MultiBody2024bfinal/Super Twisting Sliding Mode Controller/unwrap3 ==
  input_angle : Inport
  MATLAB Function1 : MATLAB Function  TreatAsAtomicUnit=on
  Memory : Memory
  unwrapped_angle : Outport
  wires:
  MATLAB Function1/1(unwrapped_angle) -> unwrapped_angle/1, Memory/1
  Memory/1 -> MATLAB Function1/2(prev_angle)
  input_angle/1 -> MATLAB Function1/1(input_angle)

== matlab function MultiBody2024bfinal/Monitoring/MATLAB Function ==
  data: u input; y output
function y = fcn(u)

y = sqrt(u'*u);

== matlab function MultiBody2024bfinal/Monitoring/MATLAB Function1 ==
  data: u input; y output
function y = fcn(u)

y = sqrt(u'*u);

== matlab function MultiBody2024bfinal/Super Twisting Sliding Mode Controller/MATLAB Function ==
  data: x input; dX output; Angle input
function dX = fcn(x,Angle)
psi = x(3);
psi0 = Angle(3);
theta0 = Angle(2);
if psi0>=-90 && psi0<=0 && theta0>0
    if abs(psi)<1*pi/180

        w = 0;
    else
        w = 1;
    end
elseif psi0<=90 && psi0>=0 && theta0>0
    if abs(psi)<1*pi/180

        w = 0;
    else
        w = -1;
    end


elseif psi0<=180 && psi0>=90 && theta0<0
    if abs(psi)>179*pi/180

        w = 0;
    else
        w = 1;
    end

elseif psi0<=-90 && psi0>=-180 && theta0<0
    if abs(psi)>179*pi/180

        w = 0;
    else
        w = -1;
    end
    
else
    w= 0;
end
dx = w * cos(psi);
dy = w * sin(psi);
dtheta = w;
dX = [dx;dy;dtheta];

== matlab function MultiBody2024bfinal/Super Twisting Sliding Mode Controller/MATLAB Function6 ==
  data: psi_m input; psi_d input; ddpsi_d input; z1 input; z2 input; z3 input; eta input; deta input; v1 input; v2 input; v_NED input; dv_NED input; v_d input; dv_d input; ddv_d input; dz1 output; eta_d input; deta_d input; ddeta_d input; z4 input; de4 input; dz2 output; dz3 output; T_theta output; param parameter; T_Left output; T_Right output; T_Up_Right output; T_Up_Left output; u1 output; T_Middle output; dz4 output; u4 output; eta_d output; e4 output; sv output; ev output
function [dz1,dz2,dz3,T_theta,T_Left,T_Right,T_Up_Right,T_Up_Left,u1,T_Middle,dz4,u4,eta_d,e4,sv,ev] = fcn(psi_m,psi_d,ddpsi_d,z1,z2,z3,eta,deta,v1,v2,v_NED,dv_NED,v_d,dv_d,ddv_d,eta_d,deta_d,ddeta_d,z4,de4,param)


phi = eta(1)*pi/180;
theta = eta(2)*pi/180;
psi = eta(3)*pi/180;

% Parametres

m = param.m ;
l_x = param.l_x ;
l_y = param.l_y ;
l_z = param.l_z ;

I_b = param.I_b;
r_g_b = param.r_g_b;
g0 =param.g0 ;

%================================================


% The equation 2.68
C_RB = [zeros(3,3) -m*S(v1)-m*S(S(v2)*r_g_b);...
    -m*S(v1)-m*S(S(v2)*r_g_b) m*S(S(v1)*r_g_b)-S(I_b*v2)];



% The equation 2.62

M_RB = [m * eye(3) -m * S(r_g_b);m * S(r_g_b) I_b];


%The equation 2.16
R_z = [cos(psi) -sin(psi) 0;sin(psi) cos(psi) 0;0 0 1];
R_y = [cos(theta) 0 sin(theta);0 1 0;-sin(theta) 0 cos(theta)];
R_x = [1 0 0;0 cos(phi) -sin(phi);0 sin(phi) cos(phi)];
R_b_n = R_z*R_y*R_x;

% The equation 4.5 in HMCH(Fossen's book)
f_g_n = [0 0 m*g0]';
g = -[R_b_n\f_g_n;S(r_g_b)*inv(R_b_n)*f_g_n];


% The equation 2.29

T_theta = [1 sin(phi) * tan(theta) cos(phi) * tan(theta);...
    0 cos(phi) -sin(phi);...
    0 sin(phi)/cos(theta) cos(phi)/cos(theta)];




%% Position Control
k1 = [20 200 100 5];
k2 = [120 300 300 5];
Lamda = diag([20.5 20 0]);
 Lamdav = 0.4;
Lamda4 = 40.1;
e4 = psi_d - psi_m;
s4 = de4 + Lamda4 * e4;

F4 = Lamda4 * de4 + ddpsi_d ;
u_bar4 = -k1(4) * sign(s4)*abs(s4)^0.5  + z4;
u4 = (u_bar4 - F4);
dz4 = -k2(4) * sign(s4)  ;

if u4>209
    u4 = 209;
end
if u4<-209
    u4 = -209;
end


%% Tilt(theta) and Bending(phi) super twisting sliding mode controller


e = eta_d - eta;
e(3) = 0;
de = deta_d - deta;
de(3) = 0;
s = de + Lamda * e ;

F = Lamda * de + ddeta_d ;


% Bending(phi) controller
u_bar1 = -k1(1) * sign(s(1))*abs(s(1))^0.5  + z1;
u1 = (u_bar1 - F(1));
% if abs(u1)<=Um1
    dz1 = -k2(1) * sign(s(1))  ;
% else
%    dz1 = -u1 ;
% 
% end


% Tilt(theta) controller
u_bar2 = -k1(2) * sign(s(2))*abs(s(2))^0.5  + z2;
u2 =(u_bar2 - F(2));
 % if abs(u2)<=Um2
    dz2 = -k2(2) * sign(s(2))  ;
 % else
 %    dz2 = -u2 ;
 % 
 % end

%Velocity controller
ev = v_d -  v_NED(3);
dev = dv_d - dv_NED(3);
sv = dev + Lamdav * ev ;

Fv = Lamdav * dev + ddv_d;% - dR_b_n * v1 - R_b_n * inv(M_RB(1:3,1:3)) *( - g(4:6))  ;
G = R_b_n * inv(M_RB(1:3,1:3));
G_inv = inv(G);
u_bar3 = -k1(3) * sign(sv(1))*abs(sv(1))^0.5  + z3;
u3 = (u_bar3 - Fv(1));
 % if abs(u3)<=Um3
  dz3 = -k2(3) * sign(sv(1))  ;
% else
%    dz3 = -u3 ;
% 
% end



%%

if u1<-209
    u1 = -209;
end
if u1>209
    u1 = 209;
end

if u1 <0
    T_Left = 209;
    T_Right = 209 + u1;
elseif u1>0
    T_Left = 209 - u1;
    T_Right = 209 ;

else
   T_Left = 209;
   T_Right = 209;
end



if u2<-209
    u2 = -209;
end
if u2>209
    u2 = 209;
end
T_Up_Right = u2+u4;
T_Up_Left = u2-u4;



T_Middle = u3;

== matlab function MultiBody2024bfinal/Super Twisting Sliding Mode Controller/MATLAB Function1 ==
  data: u input; y1 output; y2 output; Angle input; i input
function [y1,y2] = fcn(u,Angle,i)

if i>=3 && i<=4
    k = 4;
elseif i<=2
    k = 9;
else
    k = 3.5;

end
y1 = -k*u;
y2 = -sign(Angle(1))*(0.185*(abs(Angle(1))-10)+0.3)*u;

== matlab function MultiBody2024bfinal/Super Twisting Sliding Mode Controller/unwrap2/MATLAB Function1 ==
  data: input_angle input; unwrapped_angle output; prev_angle input
function unwrapped_angle = angle_unwrap(input_angle,prev_angle)
     
    if isempty(prev_angle)
        prev_angle = input_angle;
    end

    diff = input_angle - prev_angle;
    if abs(diff) > pi
        unwrapped_angle = input_angle - sign(diff) * 2 * pi;
    else
        unwrapped_angle = input_angle;
    end

end

== matlab function MultiBody2024bfinal/Super Twisting Sliding Mode Controller/MATLAB Function8 ==
  data: u input; y output
function y = fcn(u)

    y = sqrt(u'*u);

end

== matlab function MultiBody2024bfinal/Super Twisting Sliding Mode Controller/unwrap3/MATLAB Function1 ==
  data: input_angle input; unwrapped_angle output; prev_angle input
function unwrapped_angle = angle_unwrap(input_angle,prev_angle)
     
    if isempty(prev_angle)
        prev_angle = input_angle;
    end

    diff = input_angle - prev_angle;
    if abs(diff) > pi
        unwrapped_angle = input_angle - sign(diff) * 2 * pi;
    else
        unwrapped_angle = input_angle;
    end

end

== matlab function MultiBody2024bfinal/Fuel Weight Calculation and Stop Criteria/MATLAB Function1 ==
  data: int_F input; m output
function m = fcn(int_F)


g0 = 9.81;   %m/s^2; gravity acceleration
Isp = 61;   %sec; specific impulse of fuel used in CGP(in this case co2)
 

m = int_F/g0/Isp;

== matlab function MultiBody2024bfinal/Super Twisting Sliding Mode Controller/unwrap1/MATLAB Function1 ==
  data: input_angle input; unwrapped_angle output; prev_angle input
function unwrapped_angle = angle_unwrap(input_angle,prev_angle)
     
    if isempty(prev_angle)
        prev_angle = input_angle;
    end

    diff = input_angle - prev_angle;
    if abs(diff) > pi
        unwrapped_angle = input_angle - sign(diff) * 2 * pi;
    else
        unwrapped_angle = input_angle;
    end

end

== matlab function MultiBody2024bfinal/Fuel Weight Calculation and Stop Criteria/MATLAB Function2 ==
  data: u input; y output
function y = fcn(u)
if u<0.1
y = 1;
else

    y = 0;

end

== matlab function MultiBody2024bfinal/Fuel Weight Calculation and Stop Criteria/MATLAB Function3 ==
  data: u input; y output
function y = fcn(u)

y = min(u);

== matlab function MultiBody2024bfinal/Fuel Weight Calculation and Stop Criteria/MATLAB Function4 ==
  data: m_total output; m_fuel input; n_t input
function m_total = fcn(m_fuel,n_t)


%% Total weight estimation

m_equipments = 1.5;%kg

m_thrusters = n_t * 0.43;%kg
P = 300*100000;%pa
R = 8.314462618;
MM = 44 /1000;%kg/mol
T = 303.15;
V = (m_fuel * R * T/(MM * P));
Density = 568.6;%kg/m^3
m_tank = Density * V;



m_total = m_equipments + m_thrusters + m_fuel + m_tank;
end

== matlab function MultiBody2024bfinal/Fuel Weight Calculation and Stop Criteria/MATLAB Function5 ==
  data: x input; y output
function y = fcn(x)


y = sum(abs(x));
